simulink model "q_3"  (R2020a)
settings: Solver=VariableStepAuto  StartTime=0.0  StopTime=10.0  RelTol=1e-3
settings Model: Creator=Admin  LastModifiedBy=Admin

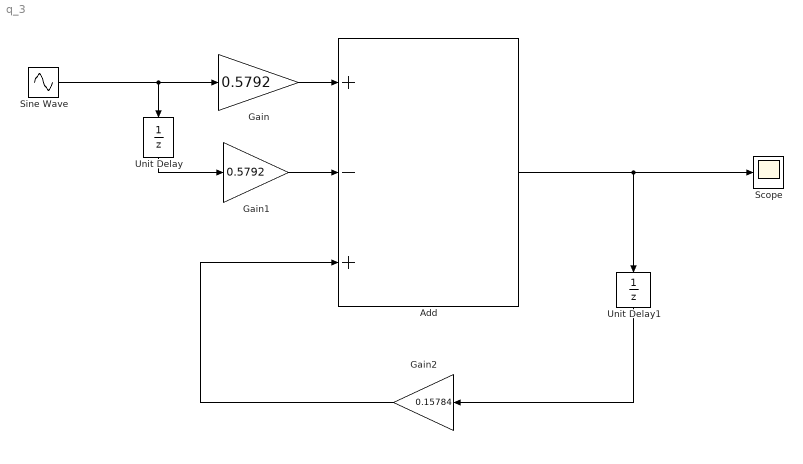
== system q_3 ==
  Add : Sum  Inputs=+-+
  Gain : Gain  Gain=0.5792
  Gain1 : Gain  Gain=0.5792
  Gain2 : Gain  Gain=0.15784
  Scope : Scope
  Sine Wave : Sin  Frequency=200*2*pi  SampleTime=0
  Unit Delay : UnitDelay  SampleTime=-1  HasFrameUpgradeWarning=on
  Unit Delay1 : UnitDelay  SampleTime=-1  HasFrameUpgradeWarning=on
  wires:
  Gain/1 -> Add/1
  Sine Wave/1 -> Unit Delay/1, Gain/1
  Gain1/1 -> Add/2
  Unit Delay/1 -> Gain1/1
  Add/1 -> Unit Delay1/1, Scope/1
  Unit Delay1/1 -> Gain2/1
  Gain2/1 -> Add/3
